simulink model "load_model"  (R2014a)
settings: Solver=ode45  StartTime=0.0  StopTime=100  RelTol=1e-3
values from neighbouring files (symbols this model uses):
  g = 9.81    [load_constants.m]
  J_drum = 1/2 * pi * w * (r_drumOuter^4 - r_drumInner^4) * rho_steel    (= 60.2097557502)    [load_constants.m]
  m_stepTotal = m_stepEach * n_step    (= 1240)    [load_constants.m]
  r_drumOuter = 0.50    (= 0.5)    [load_constants.m]
  sin_theta = sin(theta)    [load_constants.m]
settings Model: Creator=kjetibk  LastModifiedBy=kjetibk

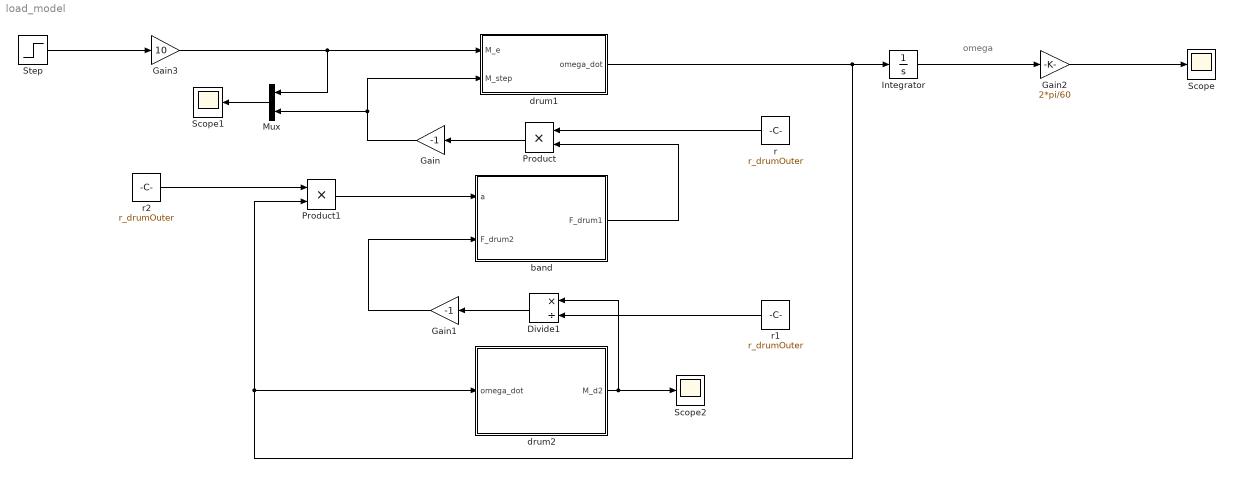
== system load_model ==
  note: omega
  Divide1 : Product  Inputs=*/
  Gain : Gain  Gain=-1
  Gain1 : Gain  Gain=-1
  Gain2 : Gain  Gain=2*pi/60
  Gain3 : Gain  Gain=10
  Integrator : Integrator
  Mux : Mux  Inputs=2
  Product : Product
  Product1 : Product
  Scope : Scope
  Scope1 : Scope
  Scope2 : Scope
      settings: SaveName=ScopeData2
  Step : Step  SampleTime=0
  band : Subsystem
  drum1 : Subsystem
  drum2 : Subsystem
  r : Constant  Value=r_drumOuter
  r1 : Constant  Value=r_drumOuter
  r2 : Constant  Value=r_drumOuter
  wires:
  Integrator/1 -> Gain2/1
  Product/1 -> Gain/1
  Step/1 -> Gain3/1
  drum1/1(omega_dot) -> Product1/2, drum2/1(omega_dot), Integrator/1
  r/1 -> Product/1
  band/1(F_drum1) -> Product/2
  drum2/1(M_d2) -> Scope2/1, Divide1/1
  r1/1 -> Divide1/2
  Divide1/1 -> Gain1/1
  Product1/1 -> band/1("a ")
  r2/1 -> Product1/1
  Gain/1 -> Mux/2, drum1/2("M_step ")
  Gain1/1 -> band/2(F_drum2)
  Gain2/1 -> Scope/1
  Mux/1 -> Scope1/1
  Gain3/1 -> Mux/1, drum1/1(M_e)

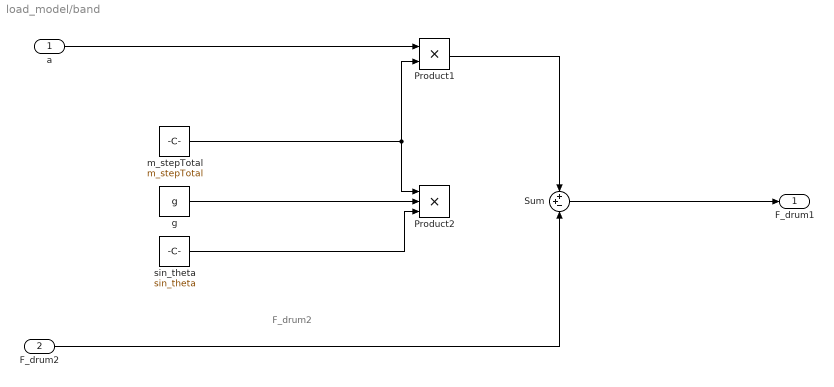
== system load_model/band ==
  note: F_drum2
  "a " : Inport
  F_drum2 : Inport  Port=2
  Product1 : Product
  Product2 : Product  Inputs=3
  Sum : Sum  Inputs=++-
  g : Constant  Value=g
  m_stepTotal : Constant  Value=m_stepTotal
  sin_theta : Constant  Value=sin_theta
  F_drum1 : Outport
  wires:
  g/1 -> Product2/2
  sin_theta/1 -> Product2/3
  F_drum2/1 -> Sum/3
  Product1/1 -> Sum/1
  "a "/1 -> Product1/1
  m_stepTotal/1 -> Product1/2, Product2/1
  Sum/1 -> F_drum1/1

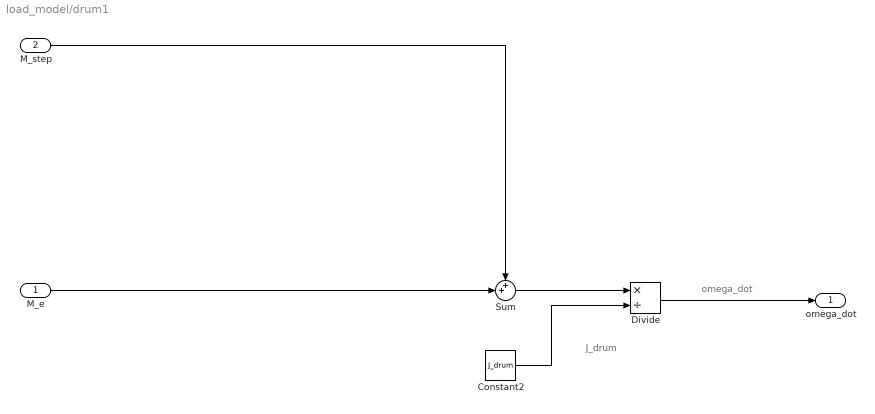
== system load_model/drum1 ==
  note: J_drum
  note: omega_dot
  M_e : Inport
  "M_step " : Inport  Port=2
  Constant2 : Constant  Value=J_drum
  Divide : Product  Inputs=*/
  Sum : Sum  Inputs=++|
  omega_dot : Outport
  wires:
  M_e/1 -> Sum/2
  "M_step "/1 -> Sum/1
  Divide/1 -> omega_dot/1
  Sum/1 -> Divide/1
  Constant2/1 -> Divide/2

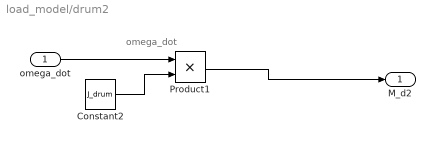
== system load_model/drum2 ==
  note: omega_dot
  omega_dot : Inport
  Constant2 : Constant  Value=J_drum
  Product1 : Product
  M_d2 : Outport
  wires:
  Constant2/1 -> Product1/2
  omega_dot/1 -> Product1/1
  Product1/1 -> M_d2/1
